simulink model "AeroModel"  (R2026b)
settings: Solver=ode45  StopTime=1
undefined symbols (not defined in the file): Aero
settings Model: DataDictionary=VehicleData.sldd  Creator=Xu Dingyi  LastModifiedBy=29358

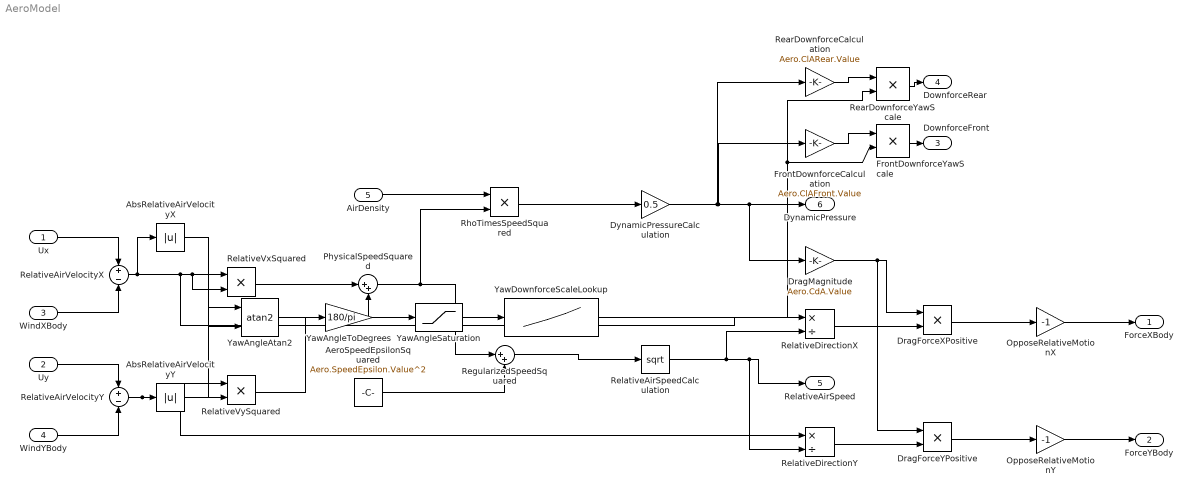
== system AeroModel ==
  Ux : Inport  OutDataTypeStr=double  PortDimensions=1
  Uy : Inport  Port=2  OutDataTypeStr=double  PortDimensions=1
  WindXBody : Inport  Port=3  OutDataTypeStr=double  PortDimensions=1
  WindYBody : Inport  Port=4  OutDataTypeStr=double  PortDimensions=1
  AirDensity : Inport  Port=5  OutDataTypeStr=double  PortDimensions=1
  AbsRelativeAirVelocityX : Abs  SaturateOnIntegerOverflow=off
  AbsRelativeAirVelocityY : Abs  SaturateOnIntegerOverflow=off
  AeroSpeedEpsilonSquared : Constant  Value=Aero.SpeedEpsilon.Value^2  OutDataTypeStr=double
  DragForceXPositive : Product  Inputs=**
  DragForceYPositive : Product  Inputs=**
  DragMagnitude : Gain  Gain=Aero.CdA.Value
  DynamicPressureCalculation : Gain  Gain=0.5
  FrontDownforceCalculation : Gain  Gain=Aero.ClAFront.Value
  FrontDownforceYawScale : Product  Inputs=**
  OpposeRelativeMotionX : Gain  Gain=-1
  OpposeRelativeMotionY : Gain  Gain=-1
  PhysicalSpeedSquared : Sum  Inputs=|++
  RearDownforceCalculation : Gain  Gain=Aero.ClARear.Value
  RearDownforceYawScale : Product  Inputs=**
  RegularizedSpeedSquared : Sum  Inputs=|++
  RelativeAirSpeedCalculation : Sqrt
  RelativeAirVelocityX : Sum  Inputs=+-
  RelativeAirVelocityY : Sum  Inputs=+-
  RelativeDirectionX : Product  Inputs=*/
  RelativeDirectionY : Product  Inputs=*/
  RelativeVxSquared : Product  Inputs=**
  RelativeVySquared : Product  Inputs=**
  RhoTimesSpeedSquared : Product  Inputs=**
  YawAngleAtan2 : Trigonometry  Operator=atan2
  YawAngleSaturation : Saturate  UpperLimit=10  LowerLimit=0
  YawAngleToDegrees : Gain  Gain=180/pi
  YawDownforceScaleLookup : Lookup_n-D  NumberOfTableDimensions=1  BreakpointsForDimension1=Aero.YawAngleGrid.Value  Table=Aero.YawDownforceScale.Value  InternalRulePriority=Speed  RndMeth=Simplest
  ForceXBody : Outport
  ForceYBody : Outport  Port=2
  DownforceFront : Outport  Port=3
  DownforceRear : Outport  Port=4
  RelativeAirSpeed : Outport  Port=5
  DynamicPressure : Outport  Port=6
  wires:
  OpposeRelativeMotionY/1 -> ForceYBody/1
  OpposeRelativeMotionX/1 -> ForceXBody/1
  DragForceYPositive/1 -> OpposeRelativeMotionY/1
  DragForceXPositive/1 -> OpposeRelativeMotionX/1
  RelativeDirectionY/1 -> DragForceYPositive/2
  RelativeDirectionX/1 -> DragForceXPositive/2
  DragMagnitude/1 -> DragForceXPositive/1, DragForceYPositive/1
  RelativeAirSpeedCalculation/1 -> RelativeDirectionY/2, RelativeAirSpeed/1, RelativeDirectionX/2
  DynamicPressureCalculation/1 -> DragMagnitude/1, DynamicPressure/1, FrontDownforceCalculation/1, RearDownforceCalculation/1
  RhoTimesSpeedSquared/1 -> DynamicPressureCalculation/1
  AirDensity/1 -> RhoTimesSpeedSquared/1
  RegularizedSpeedSquared/1 -> RelativeAirSpeedCalculation/1
  AeroSpeedEpsilonSquared/1 -> RegularizedSpeedSquared/2
  PhysicalSpeedSquared/1 -> RegularizedSpeedSquared/1, RhoTimesSpeedSquared/2
  RelativeVySquared/1 -> PhysicalSpeedSquared/2
  RelativeVxSquared/1 -> PhysicalSpeedSquared/1
  RelativeAirVelocityY/1 -> RelativeVySquared/2, RelativeDirectionY/1, RelativeVySquared/1, AbsRelativeAirVelocityY/1
  RelativeAirVelocityX/1 -> RelativeVxSquared/1, RelativeVxSquared/2, RelativeDirectionX/1, AbsRelativeAirVelocityX/1
  WindYBody/1 -> RelativeAirVelocityY/2
  Uy/1 -> RelativeAirVelocityY/1
  WindXBody/1 -> RelativeAirVelocityX/2
  Ux/1 -> RelativeAirVelocityX/1
  AbsRelativeAirVelocityY/1 -> YawAngleAtan2/1
  AbsRelativeAirVelocityX/1 -> YawAngleAtan2/2
  YawAngleAtan2/1 -> YawAngleToDegrees/1
  YawAngleToDegrees/1 -> YawAngleSaturation/1
  YawAngleSaturation/1 -> YawDownforceScaleLookup/1
  FrontDownforceCalculation/1 -> FrontDownforceYawScale/1
  RearDownforceCalculation/1 -> RearDownforceYawScale/1
  YawDownforceScaleLookup/1 -> FrontDownforceYawScale/2, RearDownforceYawScale/2
  FrontDownforceYawScale/1 -> DownforceFront/1
  RearDownforceYawScale/1 -> DownforceRear/1
